simulink model "final_fuzzy_modified_fullfuzzy"  (Simulink 7.4)
settings: Solver=ode23tb  StartTime=0.0  StopTime=0.5  MaxStep=1e-5  RelTol=1e-4
undefined symbols (not defined in the file): NEWFLC1
libraries: powerlib x25, powerlib_extras x3, fuzwiz x2, powerlib_models x1, fuzblock x1
(part 1 of 2)
settings Model: Creator=Pelab  LastModifiedBy=NEC@SATYA  SimulationMode=accelerator
settings SolverCC: ZeroCrossControl=DisableAll
settings OptimizationCC: InitFltsAndDblsToZero=on
settings DebuggingCC: SaveWithParameterizedLinksMsg=none  SignalResolutionControl=TryResolveAllWithWarning  MultiTaskDSMMsg=warning  MultiTaskCondExecSysMsg=none
settings HardwareCC: TargetEndianess=LittleEndian  TargetHWDeviceType=MATLAB Host  ProdEqTarget=off
settings RTWCC: SystemTargetFile=accel.tlc  TemplateMakefile=accel_default_tmf  ProcessScript=accel_make_rtw_hook  IncludeERTFirstTime=on
settings STFCustomTargetCC: TargetFcnLib=ansi_tfl_tmw.mat  GeneratePreprocessorConditionals=Disable all  SystemTargetFile=accel.tlc

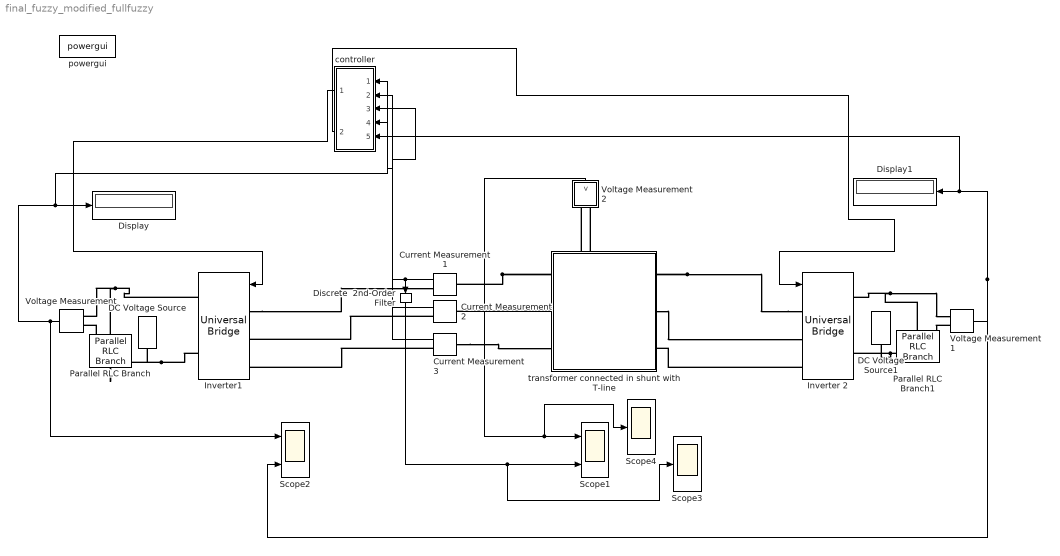
== system final_fuzzy_modified_fullfuzzy ==
  Current Measurement1 : powerlib/Measurements/Current Measurement  DialogController=POWERSYS.PowerSysDialog  SystemSampleTime=-1  PhasorSimulation=off  OutputType=Complex  PSBequivalent=0
  Current Measurement2 : powerlib/Measurements/Current Measurement  DialogController=POWERSYS.PowerSysDialog  SystemSampleTime=-1  PhasorSimulation=off  OutputType=Complex  PSBequivalent=0
  Current Measurement3 : powerlib/Measurements/Current Measurement  DialogController=POWERSYS.PowerSysDialog  SystemSampleTime=-1  PhasorSimulation=off  OutputType=Complex  PSBequivalent=0
  DC Voltage Source : powerlib/Electrical Sources/DC Voltage Source  DialogController=POWERSYS.PowerSysDialog  SystemSampleTime=-1  Amplitude=805.27  Measurements=None
  DC Voltage Source1 : powerlib/Electrical Sources/DC Voltage Source  DialogController=POWERSYS.PowerSysDialog  SystemSampleTime=-1  Amplitude=294.72  Measurements=None
  Discrete  2nd-Order Filter : powerlib_extras/Discrete  Control Blocks/Discrete  2nd-Order Filter  DialogController=POWERSYS.PowerSysDialog  SystemSampleTime=-1  FilterType=Lowpass  Fo=72  Zeta=0.707  Ts=50e-6  Initialize=off  Vac_Init=[0.8 -25 60]  Vdc_Init=-0.4  PlotResponse=off  param1=[1 500 1]
  Display : Display
      settings: Decimation=2
  Display1 : Display
  Inverter 2 : powerlib/Power Electronics/Universal Bridge  DialogController=POWERSYS.PowerSysDialog  SystemSampleTime=-1  Arms=3  SnubberResistance=1e5  SnubberCapacitance=inf  Device=Ideal Switches  Ron=1e-3  Lon=0  ForwardVoltages="[  0  0  ]"  ForwardVoltage=0  GTOparameters=[ 10e-6 , 20e-6 ]  IGBTparameters=[ 1e-6 , 2e-6 ]  Measurements=None  Measurements_2=None  converterType=Rectifier
  Inverter1 : powerlib/Power Electronics/Universal Bridge  DialogController=POWERSYS.PowerSysDialog  SystemSampleTime=-1  Arms=3  SnubberResistance=1e5  SnubberCapacitance=inf  Device=Ideal Switches  Ron=1e-3  Lon=0  ForwardVoltages="[  0  0  ]"  ForwardVoltage=0  GTOparameters=[ 10e-6 , 20e-6 ]  IGBTparameters=[ 1e-6 , 2e-6 ]  Measurements=None  Measurements_2=None  converterType=Rectifier
  Parallel RLC Branch : powerlib/Elements/Parallel RLC Branch  DialogController=POWERSYS.PowerSysDialog  PhysicalDomain=powersysdomain  SubClassName=unknown  LeftPortType=p1  RightPortType=p1  LConnTagsString=a  RConnTagsString=__new0  BranchType=RC  Resistance=1e3  Inductance=1e-3  SetiL0=off  InitialCurrent=0  Capacitance=4700e-6  Setx0=on  InitialVoltage=-805.27  Measurements=None
  Parallel RLC Branch1 : powerlib/Elements/Parallel RLC Branch  DialogController=POWERSYS.PowerSysDialog  PhysicalDomain=powersysdomain  SubClassName=unknown  LeftPortType=p1  RightPortType=p1  LConnTagsString=a  RConnTagsString=__new0  BranchType=RC  Resistance=1e3  Inductance=1e-3  SetiL0=off  InitialCurrent=0  Capacitance=4700e-6  Setx0=on  InitialVoltage=-294.72  Measurements=None
  Scope1 : Scope  NumInputPorts=2
      settings: TimeRange=0.5  YMin=-750~-100  YMax=200~40  SampleInput=on  SampleTime=1e-6
  Scope2 : Scope  NumInputPorts=2
      settings: TimeRange=0.5  YMin=0~0  YMax=1000~500  SampleInput=on  SampleTime=1e-6
  Scope3 : Scope
      settings: TimeRange=0.5  YMin=-750  YMax=200  SaveName=final_yhd_iaa  SampleInput=on  SampleTime=1e-6
  Scope4 : Scope
      settings: TimeRange=0.5  YMin=-750  YMax=200  SaveName=final_thd_Vaa  SampleInput=on  SampleTime=1e-6
  Voltage Measurement : powerlib/Measurements/Voltage Measurement  DialogController=POWERSYS.PowerSysDialog  SystemSampleTime=-1  PhasorSimulation=off  OutputType=Complex  PSBequivalent=0
  Voltage Measurement1 : powerlib/Measurements/Voltage Measurement  DialogController=POWERSYS.PowerSysDialog  SystemSampleTime=-1  PhasorSimulation=off  OutputType=Complex  PSBequivalent=0
  Voltage Measurement2 : Subsystem  AncestorBlock=powerlib/Measurements/Voltage Measurement  DialogController=POWERSYS.PowerSysDialog  mask(Voltage Measurement){PhasorSimulation=off, OutputType=Complex, PSBequivalent=0}
      mask prompts: PhasorSimulation "Phasor simulation"; OutputType "Output signal :"; PSBequivalent "Equivalent circuit"
      mask help: Ideal voltage measurement.
      mask init:
      | block = gcb;
      | powericon('psbloadfunction',block,'Measurement Block','Initialize');
      | powericon('MeasurementBlockInit',block);
      | power_initmask();
      settings: CopyFcn=powericon('psbloadfunction',gcb,'Measurement Block','UpdateGotoTag');
      mask Help: web(psbhelp);
      mask StyleString: checkbox,popup(Complex|Real-Imag|Magnitude-Angle|Magnitude),edit
  controller : Subsystem
  powergui : powerlib/powergui  SystemSampleTime=-1  SimulationMode=Continuous  SampleTime=0  frequency=60  SPID=off  DisableSnubberDevices=off  DisableRonSwitches=off  DisableVfSwitches=off  SwTol=0  Interpol=off  frequencyindice=50  echomessages=off  HookPort=off  DisplayEquations=off  FunctionMessages=off  EnableUseOfTLC=off  x0status=blocks  RestoreLinks=warning  Frange=[0:2:500]  Ylog=off  Xlog=on  ShowGrid=off  save=off  variable=ZData  structure=final_thd  ZoomFFT=off  StartTime=0.08  cycles=1  DisplayStyle=1  fundamental=50  FreqAxis=on  MaxFrequency=2500  frequencyindicesteady=1  RmsSteady=1  display=off  Ts=0  methode=off
  transformer connected in shunt with T-line : Subsystem
  wires:
  Voltage Measurement1/1 -> Display1/1, controller/5(In5), Scope2/2
  Voltage Measurement/1 -> Display/1, controller/4(In4), Scope2/1
  Current Measurement1/1 -> controller/1(In1), Discrete  2nd-Order Filter/1
  Current Measurement2/1 -> controller/2(In2)
  Current Measurement3/1 -> controller/3(In3)
  controller/1(Out1) -> Inverter1/1
  controller/2(Out2) -> Inverter 2/1
  Voltage Measurement2/1(v) -> Scope1/1, Scope4/1
  Discrete  2nd-Order Filter/1 -> Scope1/2, Scope3/1
  connections:
  Inverter1/RConn2 -- Parallel RLC Branch/LConn1 -- Voltage Measurement/LConn2 -- DC Voltage Source/LConn1
  Parallel RLC Branch1/LConn1 -- Voltage Measurement1/LConn2 -- Inverter 2/RConn2 -- DC Voltage Source1/LConn1
  Inverter 2/LConn1 -- transformer connected in shunt with T-line/LConn1 -- Voltage Measurement2/LConn2
  transformer connected in shunt with T-line/LConn2 -- Inverter 2/LConn2
  Inverter 2/LConn3 -- transformer connected in shunt with T-line/LConn3
  Parallel RLC Branch/RConn1 -- Inverter1/RConn1 -- Voltage Measurement/LConn1
  Parallel RLC Branch1/RConn1 -- Inverter 2/RConn1 -- Voltage Measurement1/LConn1
  transformer connected in shunt with T-line/RConn1 -- Current Measurement1/LConn1 -- Voltage Measurement2/LConn1
  Inverter1/LConn1 -- Current Measurement1/RConn1
  transformer connected in shunt with T-line/RConn2 -- Current Measurement2/LConn1
  Current Measurement2/RConn1 -- Inverter1/LConn2
  Current Measurement3/LConn1 -- transformer connected in shunt with T-line/RConn3
  Current Measurement3/RConn1 -- Inverter1/LConn3

== system final_fuzzy_modified_fullfuzzy/Voltage Measurement2 ==
  Discrete  2nd-Order Filter : powerlib_extras/Discrete  Control Blocks/Discrete  2nd-Order Filter  DialogController=POWERSYS.PowerSysDialog  SystemSampleTime=-1  FilterType=Lowpass  Fo=2000  Zeta=0.707  Ts=50e-6  Initialize=off  Vac_Init=[0.8 -25 60]  Vdc_Init=-0.4  PlotResponse=off  param1=[1 500 1]
  VoltageMeasurement : PMComponent  PhysicalDomain=powersysdomain  LeftPortType=p1  RightPortType=p1  LConnTagsString=+  RConnTagsString=-
      mask Type: InnerPowersysBlock
  do not delete this gain : Gain  ParameterDataType=sfix(16)  ParameterScaling=2^0  OutDataType=sfix(16)  OutScaling=2^0
  model : powerlib_models/Continuous/Measurement  SystemSampleTime=-1
  + : PMIOPort  Port=1  Side=Left
  - : PMIOPort  Port=2  Side=Left
  v : Outport  OutDataType=sfix(16)  OutScaling=2^0  InitialOutput=0
  wires:
  do not delete this gain/1 -> Discrete  2nd-Order Filter/1
  model/1 -> do not delete this gain/1
  [tpa3b51407_3347_4229_bbae_ba988a9393db] -> model/1
  Discrete  2nd-Order Filter/1 -> v/1
  connections:
  -/RConn1 -- VoltageMeasurement/RConn1
  +/RConn1 -- VoltageMeasurement/LConn1

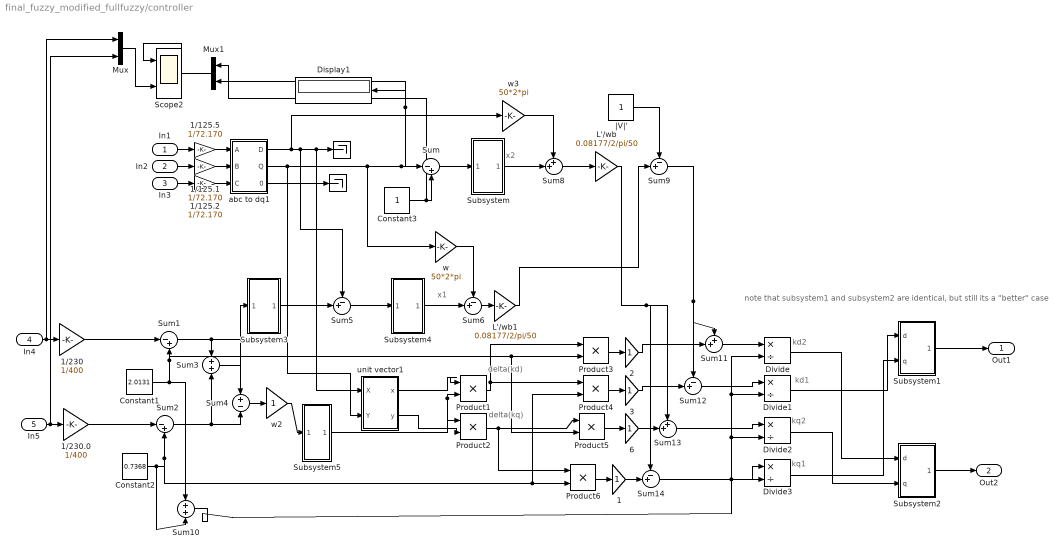
== system final_fuzzy_modified_fullfuzzy/controller ==
  note: x1
  note: x2
  note: delta(kd)
  note: delta(kq)
  note: kq2
  note: kd2
  note: kd1
  note: kq1
  note: note that subsystem1 and subsystem2 are identical,
      | but still its a "better" case
  In1 : Inport  OutDataType=sfix(16)  OutScaling=2^0
  In2 : Inport  Port=2  OutDataType=sfix(16)  OutScaling=2^0
  In3 : Inport  Port=3  OutDataType=sfix(16)  OutScaling=2^0
  In4 : Inport  Port=4  OutDataType=sfix(16)  OutScaling=2^0
  In5 : Inport  Port=5  OutDataType=sfix(16)  OutScaling=2^0
  " " : Terminator
  "  " : Terminator
  {1..3,6} (4 alike) : Gain  ParameterDataType=sfix(16)  ParameterScaling=2^0  OutDataType=sfix(16)  OutScaling=2^0
  1/125.1 : Gain  Gain=1/72.170  ParameterDataType=sfix(16)  ParameterScaling=2^0  OutDataType=sfix(16)  OutScaling=2^0
  1/125.2 : Gain  Gain=1/72.170  ParameterDataType=sfix(16)  ParameterScaling=2^0  OutDataType=sfix(16)  OutScaling=2^0
  1/125.5 : Gain  Gain=1/72.170  ParameterDataType=sfix(16)  ParameterScaling=2^0  OutDataType=sfix(16)  OutScaling=2^0
  1/230 : Gain  Gain=1/400  ParameterDataType=sfix(16)  ParameterScaling=2^0  OutDataType=sfix(16)  OutScaling=2^0
  1/230.0 : Gain  Gain=1/400  ParameterDataType=sfix(16)  ParameterScaling=2^0  OutDataType=sfix(16)  OutScaling=2^0
  Constant1 : Constant  Value=2.0131  OutDataType=sfix(16)  OutScaling=2^0
  Constant2 : Constant  Value=0.7368  OutDataType=sfix(16)  OutScaling=2^0
  Constant3 : Constant  OutDataType=sfix(16)  OutScaling=2^0
  Display1 : Display
  Divide{,1..3} (4 alike) : Product  Inputs=*/  OutDataType=sfix(16)  OutScaling=2^-10
  L'/wb : Gain  Gain=0.08177/2/pi/50  ParameterDataType=sfix(16)  ParameterScaling=2^0  OutDataType=sfix(16)  OutScaling=2^0
  L'/wb1 : Gain  Gain=0.08177/2/pi/50  ParameterDataType=sfix(16)  ParameterScaling=2^0  OutDataType=sfix(16)  OutScaling=2^0
  Mux : Mux  Inputs=2
  Mux1 : Mux  Inputs=2
  Product{1..6} (6 alike) : Product  OutDataType=sfix(16)  OutScaling=2^0  RndMeth=Zero
  Scope2 : Scope  NumInputPorts=2
      settings: TimeRange=0.03256302521008403  YMin=1~275  YMax=1.85~825  SaveName=ScopeData2  SampleTime=1e-6
  Subsystem : Subsystem
  Subsystem1 : Subsystem
  Subsystem2 : Subsystem
  Subsystem3 : Subsystem
  Subsystem4 : Subsystem
  Subsystem5 : Subsystem
  Sum : Sum  Inputs=|-+  OutDataType=sfix(16)  OutScaling=2^0
  Sum1 : Sum  Inputs=|-+  OutDataType=sfix(16)  OutScaling=2^0
  Sum10 : Sum  OutDataType=sfix(16)  OutScaling=2^0
  Sum11 : Sum  Inputs=++|  OutDataType=sfix(16)  OutScaling=2^0
  Sum{5..6,9,12,14} (5 alike) : Sum  Inputs=-+|  OutDataType=sfix(16)  OutScaling=2^0
  Sum13 : Sum  Inputs=++|  OutDataType=sfix(16)  OutScaling=2^0
  Sum2 : Sum  Inputs=|-+  OutDataType=sfix(16)  OutScaling=2^0
  Sum3 : Sum  OutDataType=sfix(16)  OutScaling=2^0
  Sum4 : Sum  Inputs=+-  OutDataType=sfix(16)  OutScaling=2^0
  Sum8 : Sum  Inputs=++|  OutDataType=sfix(16)  OutScaling=2^0
  abc to dq1 : Subsystem
  unit vector1 : Subsystem
  w : Gain  Gain=50*2*pi  ParameterDataType=sfix(16)  ParameterScaling=2^0  OutDataType=sfix(16)  OutScaling=2^0
  w2 : Gain  ParameterDataType=sfix(16)  ParameterScaling=2^0  OutDataType=sfix(16)  OutScaling=2^0
  w3 : Gain  Gain=50*2*pi  ParameterDataType=sfix(16)  ParameterScaling=2^0  OutDataType=sfix(16)  OutScaling=2^0
  |V|' : Constant  OutDataType=sfix(16)  OutScaling=2^0
  Out1 : Outport  OutDataType=sfix(16)  OutScaling=2^0
  Out2 : Outport  Port=2  OutDataType=sfix(16)  OutScaling=2^0
  wires:
  Constant3/1 -> Sum/2, Mux1/1
  abc to dq1/1(D) -> " "/1, unit vector1/1(X), Sum5/1, w3/1
  abc to dq1/3(0) -> "  "/1
  In1/1 -> 1/125.5/1
  In2/1 -> 1/125.1/1
  In3/1 -> 1/125.2/1
  In4/1 -> 1/230/1, Mux/1
  In5/1 -> 1/230.0/1, Mux/2
  Constant1/1 -> Sum1/2, Product3/2, Product5/2, Sum10/1
  Constant2/1 -> Sum2/2, Product6/2, Product4/2, Sum10/2
  Sum/1 -> Subsystem/1(In3)
  Sum1/1 -> Sum3/1, Sum4/1
  Sum2/1 -> Sum3/2, Sum4/2
  abc to dq1/2(Q) -> w/1, Sum/1, Display1/1, Mux1/2, unit vector1/2(Y)
  Sum5/1 -> Subsystem4/1(In3)
  Sum4/1 -> w2/1
  Sum3/1 -> Subsystem3/1(In3)
  Product1/1 -> Product4/1, Product3/1
  Product2/1 -> Product5/1, Product6/1
  |V|'/1 -> Sum9/1
  Sum9/1 -> Sum11/1, Sum12/1
  Sum11/1 -> Divide/1
  Sum10/1 -> Divide/2, Divide1/2, Divide2/2, Divide3/2
  Sum12/1 -> Divide1/1
  Product5/1 -> 6/1
  Sum13/1 -> Divide2/1
  Product6/1 -> 1/1
  Sum14/1 -> Divide3/1
  Sum6/1 -> L'/wb1/1
  unit vector1/1(x) -> Product1/1
  unit vector1/2(y) -> Product2/2
  Product3/1 -> 2/1
  Product4/1 -> 3/1
  Subsystem/1(Out1) -> Sum8/2
  Subsystem4/1(Out1) -> Sum6/2
  L'/wb/1 -> Sum13/1, Sum14/1
  L'/wb1/1 -> Sum9/2
  1/1 -> Sum14/2
  6/1 -> Sum13/2
  2/1 -> Sum11/2
  3/1 -> Sum12/2
  Sum8/1 -> L'/wb/1
  w2/1 -> Subsystem5/1(In3)
  Subsystem1/1(pwm) -> Out1/1
  Subsystem2/1(pwm) -> Out2/1
  Divide/1 -> Subsystem2/1(d)
  Divide1/1 -> Subsystem1/1(d)
  Divide2/1 -> Subsystem2/2(q)
  Divide3/1 -> Subsystem1/2(q)
  1/230/1 -> Sum1/1
  1/230.0/1 -> Sum2/1
  1/125.5/1 -> abc to dq1/1(A)
  1/125.1/1 -> abc to dq1/2(B)
  1/125.2/1 -> abc to dq1/3(C)
  Subsystem3/1(Out1) -> Sum5/2
  Mux/1 -> Scope2/2
  Mux1/1 -> Scope2/1
  w3/1 -> Sum8/1
  w/1 -> Sum6/1
  Subsystem5/1(Out1) -> Product1/2, Product2/1

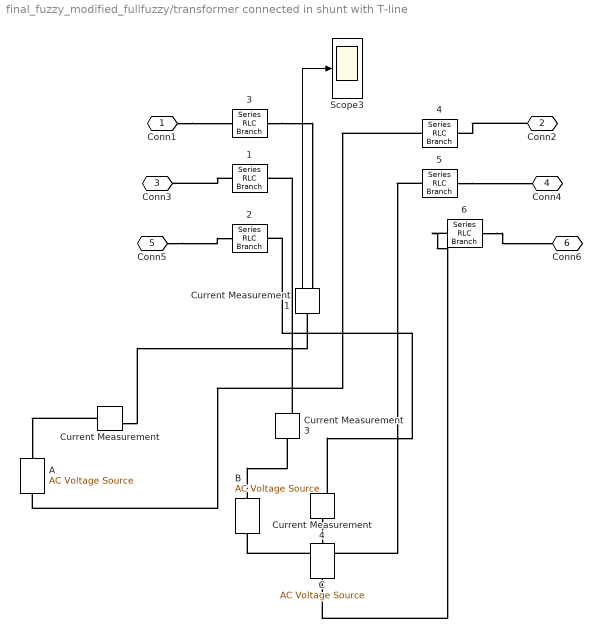
== system final_fuzzy_modified_fullfuzzy/transformer connected in shunt with T-line ==
    {1..6} (6 alike) : powerlib/Elements/Series RLC Branch  DialogController=POWERSYS.PowerSysDialog  PhysicalDomain=powersysdomain  SubClassName=unknown  LeftPortType=p1  RightPortType=p1  LConnTagsString=__new0  RConnTagsString=__new0  BranchType=RL  Resistance=0.6  Inductance=(2.5e-3)/2  SetiL0=off  InitialCurrent=0  Capacitance=1e-6  Setx0=off  InitialVoltage=0  Measurements=None
  A : powerlib/Electrical Sources/AC Voltage Source  DialogController=POWERSYS.PowerSysDialog  SystemSampleTime=-1  Amplitude=400*1.414  Phase=0  Frequency=50  SampleTime=0  Measurements=None
  B : powerlib/Electrical Sources/AC Voltage Source  DialogController=POWERSYS.PowerSysDialog  SystemSampleTime=-1  Amplitude=400*1.414  Phase=-120  Frequency=50  SampleTime=0  Measurements=None
  C : powerlib/Electrical Sources/AC Voltage Source  DialogController=POWERSYS.PowerSysDialog  SystemSampleTime=-1  Amplitude=400*1.414  Phase=-240  Frequency=50  SampleTime=0  Measurements=None
  Current Measurement{,1,3..4} (4 alike) : powerlib/Measurements/Current Measurement  DialogController=POWERSYS.PowerSysDialog  SystemSampleTime=-1  PhasorSimulation=off  OutputType=Complex  PSBequivalent=0
  Scope3 : Scope
      settings: TimeRange=0.5  YMin=-100  YMax=100  SaveName=i1  SampleInput=on  SampleTime=1e-6
  Conn1 : PMIOPort  Port=1  Side=Right
  Conn2 : PMIOPort  Port=2  Side=Left
  Conn3 : PMIOPort  Port=3  Side=Right
  Conn4 : PMIOPort  Port=4  Side=Left
  Conn5 : PMIOPort  Port=5  Side=Right
  Conn6 : PMIOPort  Port=6  Side=Left
  wires:
  Current Measurement1/1 -> Scope3/1
  connections:
  Conn1/RConn1 -- "  3"/RConn1
  "  1"/RConn1 -- Conn3/RConn1
  "  5"/LConn1 -- Conn4/RConn1
  Conn5/RConn1 -- "  2"/RConn1
  "  6"/LConn1 -- Conn6/RConn1
  Current Measurement/RConn1 -- Current Measurement1/LConn1
  "  4"/RConn1 -- A/LConn1
  "  3"/LConn1 -- Current Measurement1/RConn1
  Current Measurement4/RConn1 -- "  2"/LConn1
  Current Measurement3/RConn1 -- "  1"/LConn1
  Conn2/RConn1 -- "  4"/LConn1
  Current Measurement/LConn1 -- A/RConn1
  B/RConn1 -- Current Measurement3/LConn1
  "  5"/RConn1 -- B/LConn1
  Current Measurement4/LConn1 -- C/RConn1
  "  6"/RConn1 -- C/LConn1

== system final_fuzzy_modified_fullfuzzy/controller/Subsystem ==
  In3 : Inport
  Derivative : Derivative
  Fuzzy Logic  Controller : fuzblock/Fuzzy Logic  Controller  SystemSampleTime=-1  fis=NEWFLC1
  Mux2 : Mux  Inputs=2
  Out1 : Outport
  wires:
  Mux2/1 -> Fuzzy Logic  Controller/1
  In3/1 -> Mux2/1, Derivative/1
  Fuzzy Logic  Controller/1 -> Out1/1
  Derivative/1 -> Mux2/2

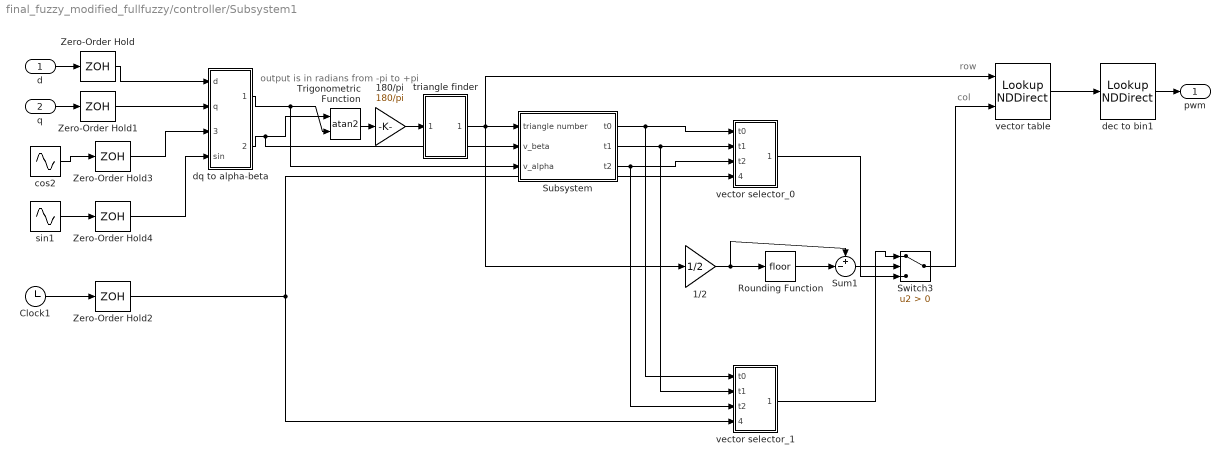
== system final_fuzzy_modified_fullfuzzy/controller/Subsystem1 ==
  note: output is in radians from -pi to +pi
  note: col
  note: row
  d : Inport  OutDataType=sfix(16)  OutScaling=2^0
  q : Inport  Port=2  OutDataType=sfix(16)  OutScaling=2^0
  1/2 : Gain  Gain=1/2  ParameterDataType=sfix(16)  ParameterScaling=2^0  OutDataType=sfix(16)  OutScaling=2^0
  180/pi : Gain  Gain=180/pi  ParameterDataType=sfix(16)  ParameterScaling=2^0  OutDataType=sfix(16)  OutScaling=2^0
  Clock1 : Clock
      settings: Decimation=10
  Rounding Function : Rounding
  Subsystem : Subsystem
  Sum1 : Sum  Inputs=+-|  OutDataType=sfix(16)  OutScaling=2^0
  Switch3 : Switch  Criteria=u2 > Threshold
  Trigonometric Function : Trigonometry  Operator=atan2
  Zero-Order Hold{,1..4} (5 alike) : ZeroOrderHold  SampleTime=(20e-3)/18
  cos2 : Sin  Amplitude=1  Bias=0  Frequency=50*2*pi  Phase=pi/2  Samples=10  SampleTime=0  Offset=0
  dec to bin1 : LookupNDDirect  InputsSelectThisObjectFromTable=Column  Table=[0 1 1 0 0 0 1 1; 1 0 0 1 1 1 0 0; 0 0 1 1 1 0 0 1; 1 1 0 0 0 1 1 0; 0 0 0 0 1 1 1 1; 1 1 1 1 0 0 0 0]
  dq to alpha-beta : Subsystem
  sin1 : Sin  Amplitude=1  Bias=0  Frequency=50*2*pi  Phase=0  Samples=10  SampleTime=0  Offset=0
  triangle finder : Subsystem
  vector selector_0 : Subsystem
  vector selector_1 : Subsystem
  vector table : LookupNDDirect  Table=[0 5 6 7 6 5 0; 0 1 6 7 6 1 0; 0 1 2 7 2 1 0; 0 3 2 7 2 3 0; 0 3 4 7 4 3 0; 0 5 4 7 4 5 0]
  pwm : Outport  OutDataType=sfix(16)  OutScaling=2^0
  wires:
  dq to alpha-beta/2(beta) -> Trigonometric Function/1, Subsystem/2(v_beta)
  dq to alpha-beta/1(alpha) -> Trigonometric Function/2, Subsystem/3(v_alpha)
  Trigonometric Function/1 -> 180/pi/1
  180/pi/1 -> triangle finder/1(In1)
  triangle finder/1(Out1) -> Subsystem/1(triangle number), vector table/1, 1/2/1
  Zero-Order Hold/1 -> dq to alpha-beta/1(d)
  Zero-Order Hold1/1 -> dq to alpha-beta/2(q)
  Clock1/1 -> Zero-Order Hold2/1
  Zero-Order Hold2/1 -> vector selector_0/4(hold_time), vector selector_1/4(hold_time)
  vector table/1 -> dec to bin1/1
  dec to bin1/1 -> pwm/1
  d/1 -> Zero-Order Hold/1
  q/1 -> Zero-Order Hold1/1
  cos2/1 -> Zero-Order Hold3/1
  Zero-Order Hold3/1 -> dq to alpha-beta/3(cos)
  sin1/1 -> Zero-Order Hold4/1
  Zero-Order Hold4/1 -> dq to alpha-beta/4(sin)
  1/2/1 -> Rounding Function/1, Sum1/1
  Rounding Function/1 -> Sum1/2
  Sum1/1 -> Switch3/2
  Subsystem/1(t0) -> vector selector_0/1(t0), vector selector_1/1(t0)
  Subsystem/2(t1) -> vector selector_0/2(t1), vector selector_1/2(t1)
  Subsystem/3(t2) -> vector selector_0/3(t2), vector selector_1/3(t2)
  vector selector_0/1(Out1) -> Switch3/3
  Switch3/1 -> vector table/2
  vector selector_1/1(Out1) -> Switch3/1

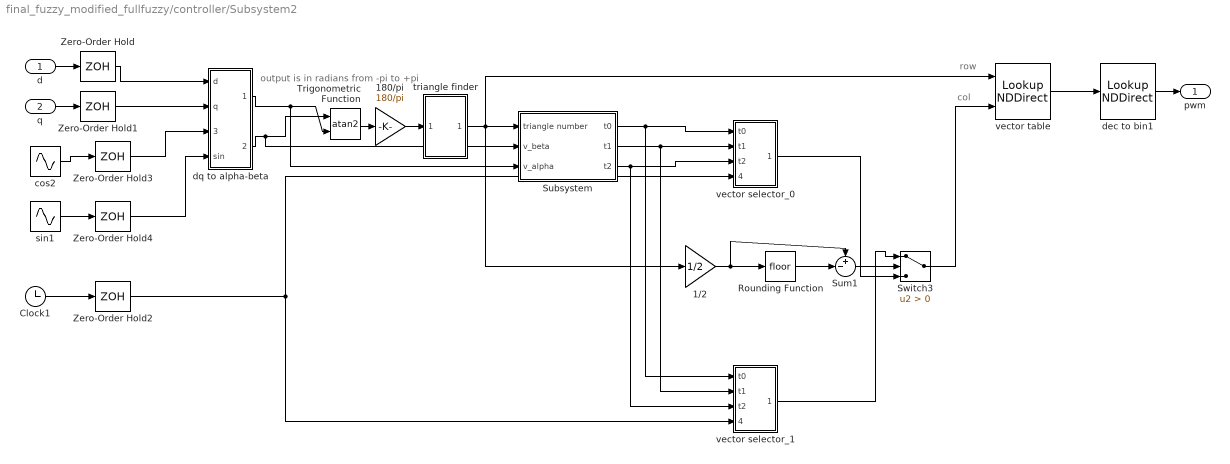
== system final_fuzzy_modified_fullfuzzy/controller/Subsystem2 ==
  note: row
  note: col
  note: output is in radians from -pi to +pi
  d : Inport  OutDataType=sfix(16)  OutScaling=2^0
  q : Inport  Port=2  OutDataType=sfix(16)  OutScaling=2^0
  1/2 : Gain  Gain=1/2  ParameterDataType=sfix(16)  ParameterScaling=2^0  OutDataType=sfix(16)  OutScaling=2^0
  180/pi : Gain  Gain=180/pi  ParameterDataType=sfix(16)  ParameterScaling=2^0  OutDataType=sfix(16)  OutScaling=2^0
  Clock1 : Clock
      settings: Decimation=10
  Rounding Function : Rounding
  Subsystem : Subsystem
  Sum1 : Sum  Inputs=+-|  OutDataType=sfix(16)  OutScaling=2^0
  Switch3 : Switch  Criteria=u2 > Threshold
  Trigonometric Function : Trigonometry  Operator=atan2
  Zero-Order Hold{,1..4} (5 alike) : ZeroOrderHold  SampleTime=(20e-3)/18
  cos2 : Sin  Amplitude=1  Bias=0  Frequency=50*2*pi  Phase=pi/2  Samples=10  SampleTime=0  Offset=0
  dec to bin1 : LookupNDDirect  InputsSelectThisObjectFromTable=Column  Table=[0 1 1 0 0 0 1 1; 1 0 0 1 1 1 0 0; 0 0 1 1 1 0 0 1; 1 1 0 0 0 1 1 0; 0 0 0 0 1 1 1 1; 1 1 1 1 0 0 0 0]
  dq to alpha-beta : Subsystem
  sin1 : Sin  Amplitude=1  Bias=0  Frequency=50*2*pi  Phase=0  Samples=10  SampleTime=0  Offset=0
  triangle finder : Subsystem
  vector selector_0 : Subsystem
  vector selector_1 : Subsystem
  vector table : LookupNDDirect  Table=[0 5 6 7 6 5 0; 0 1 6 7 6 1 0; 0 1 2 7 2 1 0; 0 3 2 7 2 3 0; 0 3 4 7 4 3 0; 0 5 4 7 4 5 0]
  pwm : Outport  OutDataType=sfix(16)  OutScaling=2^0
  wires:
  vector selector_1/1(Out1) -> Switch3/1
  Switch3/1 -> vector table/2
  vector selector_0/1(Out1) -> Switch3/3
  Subsystem/3(t2) -> vector selector_1/3(t2), vector selector_0/3(t2)
  Subsystem/2(t1) -> vector selector_1/2(t1), vector selector_0/2(t1)
  Subsystem/1(t0) -> vector selector_1/1(t0), vector selector_0/1(t0)
  Sum1/1 -> Switch3/2
  Rounding Function/1 -> Sum1/2
  1/2/1 -> Sum1/1, Rounding Function/1
  Zero-Order Hold4/1 -> dq to alpha-beta/4(sin)
  sin1/1 -> Zero-Order Hold4/1
  Zero-Order Hold3/1 -> dq to alpha-beta/3(cos)
  cos2/1 -> Zero-Order Hold3/1
  q/1 -> Zero-Order Hold1/1
  d/1 -> Zero-Order Hold/1
  dec to bin1/1 -> pwm/1
  vector table/1 -> dec to bin1/1
  Zero-Order Hold2/1 -> vector selector_1/4(hold_time), vector selector_0/4(hold_time)
  Clock1/1 -> Zero-Order Hold2/1
  Zero-Order Hold1/1 -> dq to alpha-beta/2(q)
  Zero-Order Hold/1 -> dq to alpha-beta/1(d)
  triangle finder/1(Out1) -> 1/2/1, vector table/1, Subsystem/1(triangle number)
  180/pi/1 -> triangle finder/1(In1)
  Trigonometric Function/1 -> 180/pi/1
  dq to alpha-beta/1(alpha) -> Subsystem/3(v_alpha), Trigonometric Function/2
  dq to alpha-beta/2(beta) -> Subsystem/2(v_beta), Trigonometric Function/1

== system final_fuzzy_modified_fullfuzzy/controller/Subsystem3 ==
  In3 : Inport
  Derivative : Derivative
  Fuzzy Logic  Controller : Subsystem  AncestorBlock="fuzblock/Fuzzy Logic  Controller"  mask(FIS){fis=NEWFLC1}
      mask prompts: fis "FIS file or structure:"
      mask help: FIS
      mask init:
      | fis = fuzblockmask(gcb,fis);
      mask Help: helpview([docroot '\toolbox\fuzzy\fuzzylogiccontroller.html'])
      mask Display: plot(0, -0.3, 6, -0.3, 0, 1.2, 6, 1.2, [0 6], [0 0], [1 2 3],[0 1 0],[2 3 4],[0 1 0],[3 4 5],[0 1 0])
  Mux2 : Mux  Inputs=2
  Out1 : Outport
  wires:
  Derivative/1 -> Mux2/2
  Fuzzy Logic  Controller/1(Out1) -> Out1/1
  In3/1 -> Derivative/1, Mux2/1
  Mux2/1 -> Fuzzy Logic  Controller/1(In1)

== system final_fuzzy_modified_fullfuzzy/controller/Subsystem4 ==
  In3 : Inport
  Derivative : Derivative
  Fuzzy Logic  Controller : Subsystem  AncestorBlock="fuzblock/Fuzzy Logic  Controller"  mask(FIS){fis=NEWFLC1}
      mask prompts: fis "FIS file or structure:"
      mask help: FIS
      mask init:
      | fis = fuzblockmask(gcb,fis);
      mask Help: helpview([docroot '\toolbox\fuzzy\fuzzylogiccontroller.html'])
      mask Display: plot(0, -0.3, 6, -0.3, 0, 1.2, 6, 1.2, [0 6], [0 0], [1 2 3],[0 1 0],[2 3 4],[0 1 0],[3 4 5],[0 1 0])
  Mux2 : Mux  Inputs=2
  Out1 : Outport
  wires:
  Mux2/1 -> Fuzzy Logic  Controller/1(In1)
  In3/1 -> Mux2/1, Derivative/1
  Fuzzy Logic  Controller/1(Out1) -> Out1/1
  Derivative/1 -> Mux2/2

== system final_fuzzy_modified_fullfuzzy/controller/Subsystem5 ==
  In3 : Inport
  Derivative : Derivative
  Fuzzy Logic  Controller : Subsystem  AncestorBlock="fuzblock/Fuzzy Logic  Controller"  mask(FIS){fis=NEWFLC1}
      mask prompts: fis "FIS file or structure:"
      mask help: FIS
      mask init:
      | fis = fuzblockmask(gcb,fis);
      mask Help: helpview([docroot '\toolbox\fuzzy\fuzzylogiccontroller.html'])
      mask Display: plot(0, -0.3, 6, -0.3, 0, 1.2, 6, 1.2, [0 6], [0 0], [1 2 3],[0 1 0],[2 3 4],[0 1 0],[3 4 5],[0 1 0])
  Mux2 : Mux  Inputs=2
  Out1 : Outport
  wires:
  Mux2/1 -> Fuzzy Logic  Controller/1(In1)
  In3/1 -> Mux2/1, Derivative/1
  Fuzzy Logic  Controller/1(Out1) -> Out1/1
  Derivative/1 -> Mux2/2

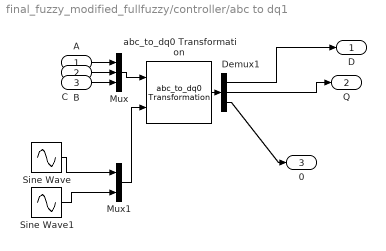
== system final_fuzzy_modified_fullfuzzy/controller/abc to dq1 ==
  A : Inport  OutDataType=sfix(16)  OutScaling=2^0
  B : Inport  Port=2  OutDataType=sfix(16)  OutScaling=2^0
  C : Inport  Port=3  OutDataType=sfix(16)  OutScaling=2^0
  Demux1 : Demux  Outputs=3
  Mux : Mux  Inputs=3
  Mux1 : Mux  Inputs=2
  Sine Wave : Sin  Amplitude=1  Bias=0  Frequency=50*2*pi  Phase=0  Samples=10  SampleTime=0  Offset=0
  Sine Wave1 : Sin  Amplitude=1  Bias=0  Frequency=50*2*pi  Phase=pi/2  Samples=10  SampleTime=0  Offset=0
  abc_to_dq0 Transformation : powerlib_extras/Measurements/abc_to_dq0 Transformation  DialogController=POWERSYS.PowerSysDialog  SystemSampleTime=-1
  D : Outport  OutDataType=sfix(16)  OutScaling=2^0
  Q : Outport  Port=2  OutDataType=sfix(16)  OutScaling=2^0
  0 : Outport  Port=3  OutDataType=sfix(16)  OutScaling=2^0
  wires:
  Demux1/3 -> 0/1
  C/1 -> Mux/3
  B/1 -> Mux/2
  A/1 -> Mux/1
  Mux/1 -> abc_to_dq0 Transformation/1
  Sine Wave/1 -> Mux1/1
  Sine Wave1/1 -> Mux1/2
  Mux1/1 -> abc_to_dq0 Transformation/2
  abc_to_dq0 Transformation/1 -> Demux1/1
  Demux1/1 -> D/1
  Demux1/2 -> Q/1

== system final_fuzzy_modified_fullfuzzy/controller/unit vector1 ==
  X : Inport  OutDataType=sfix(16)  OutScaling=2^0
  Y : Inport  Port=2  OutDataType=sfix(16)  OutScaling=2^0
  Add : Sum  OutDataType=sfix(16)  OutScaling=2^-10
  Divide : Product  Inputs=*/  OutDataType=sfix(16)  OutScaling=2^-10
  Divide1 : Product  Inputs=*/  OutDataType=sfix(16)  OutScaling=2^-10
  Math Function : Math  Operator=sqrt  OutDataType=sfix(16)  OutScaling=2^0  SaturateOnIntegerOverflow=on
  Product : Product  OutDataType=sfix(16)  OutScaling=2^0  RndMeth=Zero
  Product1 : Product  OutDataType=sfix(16)  OutScaling=2^0  RndMeth=Zero
  Saturation : Saturate  UpperLimit=inf  LowerLimit=0.0001
  x : Outport  OutDataType=sfix(16)  OutScaling=2^0
  y : Outport  Port=2  OutDataType=sfix(16)  OutScaling=2^0
  wires:
  Saturation/1 -> Divide1/2, Divide/2
  Divide1/1 -> y/1
  Divide/1 -> x/1
  Math Function/1 -> Saturation/1
  Add/1 -> Math Function/1
  Y/1 -> Divide1/1, Product1/2, Product1/1
  X/1 -> Divide/1, Product/2, Product/1
  Product1/1 -> Add/2
  Product/1 -> Add/1

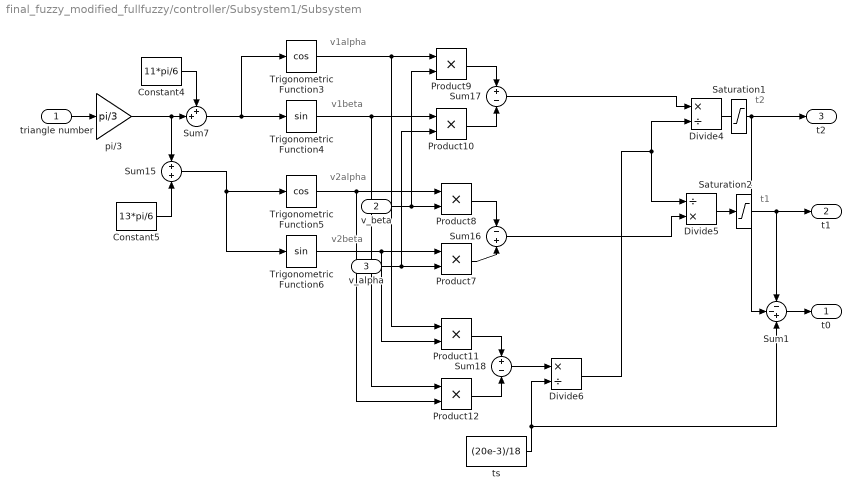
== system final_fuzzy_modified_fullfuzzy/controller/Subsystem1/Subsystem ==
  note: v1alpha
  note: v1beta
  note: v2alpha
  note: v2beta
  note: t1
  note: t2
  triangle number : Inport  OutDataType=sfix(16)  OutScaling=2^0
  v_beta : Inport  Port=2  OutDataType=sfix(16)  OutScaling=2^0
  v_alpha : Inport  Port=3  OutDataType=sfix(16)  OutScaling=2^0
  Constant4 : Constant  Value=11*pi/6  OutDataType=sfix(16)  OutScaling=2^0
  Constant5 : Constant  Value=13*pi/6  OutDataType=sfix(16)  OutScaling=2^0
  Divide4 : Product  Inputs=*/  OutDataType=sfix(16)  OutScaling=2^-10
  Divide5 : Product  Inputs=/*  OutDataType=sfix(16)  OutScaling=2^-10
  Divide6 : Product  Inputs=*/  OutDataType=sfix(16)  OutScaling=2^-10
  Product{7..12} (6 alike) : Product  OutDataType=sfix(16)  OutScaling=2^0  RndMeth=Zero
  Saturation1 : Saturate  UpperLimit=inf  LowerLimit=0
  Saturation2 : Saturate  UpperLimit=inf  LowerLimit=0
  Sum1 : Sum  Inputs=--+  OutDataType=sfix(16)  OutScaling=2^0
  Sum15 : Sum  OutDataType=sfix(16)  OutScaling=2^0
  Sum16 : Sum  Inputs=-+  OutDataType=sfix(16)  OutScaling=2^0
  Sum17 : Sum  Inputs=+-  OutDataType=sfix(16)  OutScaling=2^0
  Sum18 : Sum  Inputs=+-  OutDataType=sfix(16)  OutScaling=2^0
  Sum7 : Sum  Inputs=++|  OutDataType=sfix(16)  OutScaling=2^0
  Trigonometric Function3 : Trigonometry  Operator=cos
  Trigonometric Function4 : Trigonometry
  Trigonometric Function5 : Trigonometry  Operator=cos
  Trigonometric Function6 : Trigonometry
  pi/3 : Gain  Gain=pi/3  ParameterDataType=sfix(16)  ParameterScaling=2^0  OutDataType=sfix(16)  OutScaling=2^0
  ts : Constant  Value=(20e-3)/18  OutDataType=sfix(16)  OutScaling=2^0
  t0 : Outport  OutDataType=sfix(16)  OutScaling=2^0
  t1 : Outport  Port=2  OutDataType=sfix(16)  OutScaling=2^0
  t2 : Outport  Port=3  OutDataType=sfix(16)  OutScaling=2^0
  wires:
  Sum7/1 -> Trigonometric Function3/1, Trigonometric Function4/1
  Constant4/1 -> Sum7/1
  pi/3/1 -> Sum7/2, Sum15/1
  Constant5/1 -> Sum15/2
  Trigonometric Function5/1 -> Product8/1, Product12/2
  Trigonometric Function6/1 -> Product7/1, Product11/2
  Sum15/1 -> Trigonometric Function5/1, Trigonometric Function6/1
  Product7/1 -> Sum16/2
  Product8/1 -> Sum16/1
  Sum16/1 -> Divide5/2
  Trigonometric Function3/1 -> Product9/1, Product11/1
  Trigonometric Function4/1 -> Product10/1, Product12/1
  Product9/1 -> Sum17/1
  Product10/1 -> Sum17/2
  Sum17/1 -> Divide4/1
  Product11/1 -> Sum18/1
  Product12/1 -> Sum18/2
  Sum18/1 -> Divide6/1
  Divide6/1 -> Divide4/2, Divide5/1
  ts/1 -> Divide6/2, Sum1/3
  v_beta/1 -> Product8/2, Product9/2
  v_alpha/1 -> Product7/2, Product10/2
  Divide4/1 -> Sum1/2, t2/1
  triangle number/1 -> pi/3/1
  Divide5/1 -> Saturation2/1
  Sum1/1 -> t0/1
  Saturation2/1 -> t1/1, Sum1/1

== system final_fuzzy_modified_fullfuzzy/controller/Subsystem1/dq to alpha-beta ==
  d : Inport  OutDataType=sfix(16)  OutScaling=2^0
  q : Inport  Port=2  OutDataType=sfix(16)  OutScaling=2^0
  cos : Inport  Port=3  OutDataType=sfix(16)  OutScaling=2^0
  sin : Inport  Port=4  OutDataType=sfix(16)  OutScaling=2^0
  Product{,1..3} (4 alike) : Product  OutDataType=sfix(16)  OutScaling=2^0  RndMeth=Zero
  Sum : Sum  Inputs=+-  OutDataType=sfix(16)  OutScaling=2^0
  Sum1 : Sum  OutDataType=sfix(16)  OutScaling=2^0
  alpha : Outport  OutDataType=sfix(16)  OutScaling=2^0
  beta : Outport  Port=2  OutDataType=sfix(16)  OutScaling=2^0
  wires:
  d/1 -> Product/1, Product2/1
  q/1 -> Product1/2, Product3/1
  Product/1 -> Sum/1
  Product1/1 -> Sum/2
  Sum/1 -> alpha/1
  Product2/1 -> Sum1/1
  Product3/1 -> Sum1/2
  Sum1/1 -> beta/1
  cos/1 -> Product/2, Product3/2
  sin/1 -> Product1/1, Product2/2

== system final_fuzzy_modified_fullfuzzy/controller/Subsystem1/triangle finder ==
  In1 : Inport  OutDataType=sfix(16)  OutScaling=2^0
  4 : Gain  Gain=1/60  ParameterDataType=sfix(16)  ParameterScaling=2^0  OutDataType=sfix(16)  OutScaling=2^0
  Rounding Function : Rounding
  Sum15 : Sum  Inputs=|++  OutDataType=sfix(16)  OutScaling=2^0
  Sum7 : Sum  Inputs=|++  OutDataType=sfix(16)  OutScaling=2^0
  Switch : Switch  Criteria=u2 > Threshold  Threshold=-1
  |V|3 : Constant  Value=30  OutDataType=sfix(16)  OutScaling=2^0
  |V|4 : Constant  Value=6  OutDataType=sfix(16)  OutScaling=2^0
  Out1 : Outport  OutDataType=sfix(16)  OutScaling=2^0
  wires:
  |V|3/1 -> Sum7/2
  Sum7/1 -> 4/1
  4/1 -> Rounding Function/1
  Rounding Function/1 -> Switch/2, Switch/1, Sum15/1
  |V|4/1 -> Sum15/2
  Sum15/1 -> Switch/3
  In1/1 -> Sum7/1
  Switch/1 -> Out1/1

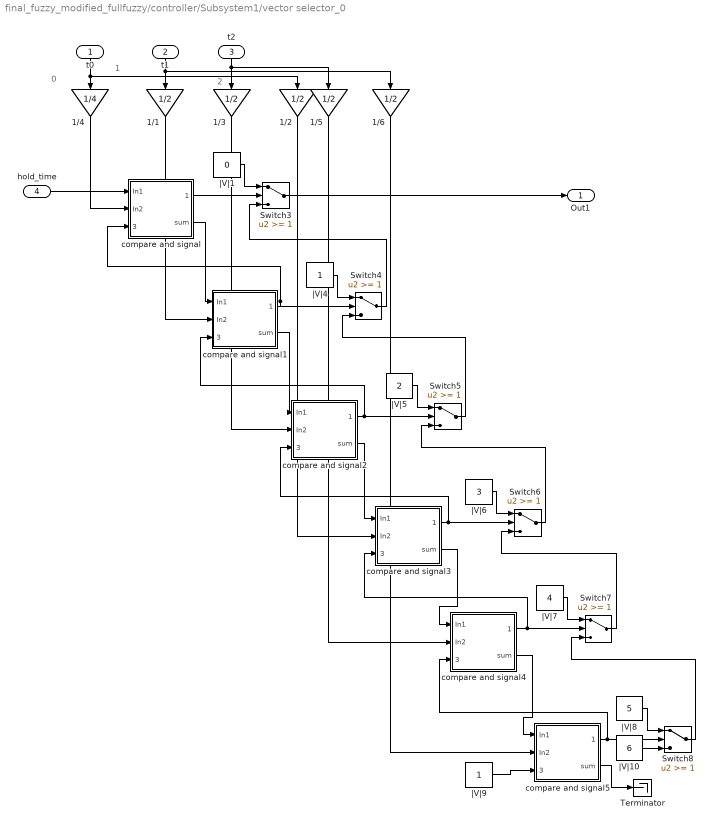
== system final_fuzzy_modified_fullfuzzy/controller/Subsystem1/vector selector_0 ==
  note: 0
  note: 1
  note: 2
  t0 : Inport
  t1 : Inport  Port=2
  t2 : Inport  Port=3
  hold_time : Inport  Port=4
  1/{1..3,5..6} (5 alike) : Gain  Gain=1/2  ParameterDataType=sfix(16)  ParameterScaling=2^0  OutDataType=sfix(16)  OutScaling=2^0
  1/4 : Gain  Gain=1/4  ParameterDataType=sfix(16)  ParameterScaling=2^0  OutDataType=sfix(16)  OutScaling=2^0
  Switch{3..8} (6 alike) : Switch  Threshold=1
  Terminator : Terminator
  compare and signal : Subsystem
  compare and signal1 : Subsystem
  compare and signal2 : Subsystem
  compare and signal3 : Subsystem
  compare and signal4 : Subsystem
  compare and signal5 : Subsystem
  |V|1 : Constant  Value=0  OutDataType=sfix(16)  OutScaling=2^0
  |V|10 : Constant  Value=6  OutDataType=sfix(16)  OutScaling=2^0
  |V|4 : Constant  OutDataType=sfix(16)  OutScaling=2^0
  |V|5 : Constant  Value=2  OutDataType=sfix(16)  OutScaling=2^0
  |V|6 : Constant  Value=3  OutDataType=sfix(16)  OutScaling=2^0
  |V|7 : Constant  Value=4  OutDataType=sfix(16)  OutScaling=2^0
  |V|8 : Constant  Value=5  OutDataType=sfix(16)  OutScaling=2^0
  |V|9 : Constant  OutDataType=sfix(16)  OutScaling=2^0
  Out1 : Outport
  wires:
  1/4/1 -> compare and signal/2(In2)
  t1/1 -> 1/1/1, 1/6/1
  t2/1 -> 1/3/1, 1/5/1
  t0/1 -> 1/4/1, 1/2/1
  hold_time/1 -> compare and signal/1(In1)
  compare and signal/1(logic_out) -> Switch3/2
  |V|1/1 -> Switch3/1
  compare and signal1/1(logic_out) -> compare and signal/3(logic_in), Switch4/2
  compare and signal/2(sum) -> compare and signal1/1(In1)
  1/1/1 -> compare and signal1/2(In2)
  |V|4/1 -> Switch4/1
  compare and signal1/2(sum) -> compare and signal2/1(In1)
  1/3/1 -> compare and signal2/2(In2)
  |V|5/1 -> Switch5/1
  compare and signal2/1(logic_out) -> Switch5/2, compare and signal1/3(logic_in)
  compare and signal2/2(sum) -> compare and signal3/1(In1)
  1/2/1 -> compare and signal3/2(In2)
  |V|6/1 -> Switch6/1
  compare and signal3/1(logic_out) -> Switch6/2, compare and signal2/3(logic_in)
  compare and signal3/2(sum) -> compare and signal4/1(In1)
  1/5/1 -> compare and signal4/2(In2)
  |V|7/1 -> Switch7/1
  compare and signal4/1(logic_out) -> Switch7/2, compare and signal3/3(logic_in)
  1/6/1 -> compare and signal5/2(In2)
  compare and signal4/2(sum) -> compare and signal5/1(In1)
  |V|8/1 -> Switch8/1
  compare and signal5/1(logic_out) -> Switch8/2, compare and signal4/3(logic_in)
  |V|9/1 -> compare and signal5/3(logic_in)
  |V|10/1 -> Switch8/3
  compare and signal5/2(sum) -> Terminator/1
  Switch8/1 -> Switch7/3
  Switch7/1 -> Switch6/3
  Switch6/1 -> Switch5/3
  Switch5/1 -> Switch4/3
  Switch4/1 -> Switch3/3
  Switch3/1 -> Out1/1

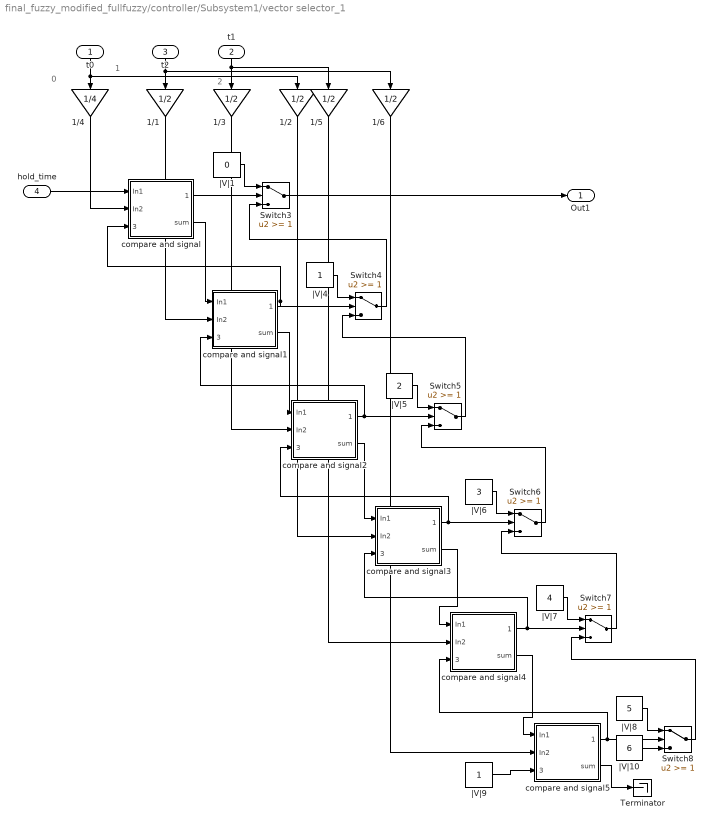
== system final_fuzzy_modified_fullfuzzy/controller/Subsystem1/vector selector_1 ==
  note: 2
  note: 1
  note: 0
  t0 : Inport
  t1 : Inport  Port=2
  t2 : Inport  Port=3
  hold_time : Inport  Port=4
  1/{1..3,5..6} (5 alike) : Gain  Gain=1/2  ParameterDataType=sfix(16)  ParameterScaling=2^0  OutDataType=sfix(16)  OutScaling=2^0
  1/4 : Gain  Gain=1/4  ParameterDataType=sfix(16)  ParameterScaling=2^0  OutDataType=sfix(16)  OutScaling=2^0
  Switch{3..8} (6 alike) : Switch  Threshold=1
  Terminator : Terminator
  compare and signal : Subsystem
  compare and signal1 : Subsystem
  compare and signal2 : Subsystem
  compare and signal3 : Subsystem
  compare and signal4 : Subsystem
  compare and signal5 : Subsystem
  |V|1 : Constant  Value=0  OutDataType=sfix(16)  OutScaling=2^0
  |V|10 : Constant  Value=6  OutDataType=sfix(16)  OutScaling=2^0
  |V|4 : Constant  OutDataType=sfix(16)  OutScaling=2^0
  |V|5 : Constant  Value=2  OutDataType=sfix(16)  OutScaling=2^0
  |V|6 : Constant  Value=3  OutDataType=sfix(16)  OutScaling=2^0
  |V|7 : Constant  Value=4  OutDataType=sfix(16)  OutScaling=2^0
  |V|8 : Constant  Value=5  OutDataType=sfix(16)  OutScaling=2^0
  |V|9 : Constant  OutDataType=sfix(16)  OutScaling=2^0
  Out1 : Outport
  wires:
  Switch3/1 -> Out1/1
  Switch4/1 -> Switch3/3
  Switch5/1 -> Switch4/3
  Switch6/1 -> Switch5/3
  Switch7/1 -> Switch6/3
  Switch8/1 -> Switch7/3
  compare and signal5/2(sum) -> Terminator/1
  |V|10/1 -> Switch8/3
  |V|9/1 -> compare and signal5/3(logic_in)
  compare and signal5/1(logic_out) -> compare and signal4/3(logic_in), Switch8/2
  |V|8/1 -> Switch8/1
  compare and signal4/2(sum) -> compare and signal5/1(In1)
  1/6/1 -> compare and signal5/2(In2)
  compare and signal4/1(logic_out) -> compare and signal3/3(logic_in), Switch7/2
  |V|7/1 -> Switch7/1
  1/5/1 -> compare and signal4/2(In2)
  compare and signal3/2(sum) -> compare and signal4/1(In1)
  compare and signal3/1(logic_out) -> compare and signal2/3(logic_in), Switch6/2
  |V|6/1 -> Switch6/1
  1/2/1 -> compare and signal3/2(In2)
  compare and signal2/2(sum) -> compare and signal3/1(In1)
  compare and signal2/1(logic_out) -> compare and signal1/3(logic_in), Switch5/2
  |V|5/1 -> Switch5/1
  1/3/1 -> compare and signal2/2(In2)
  compare and signal1/2(sum) -> compare and signal2/1(In1)
  |V|4/1 -> Switch4/1
  1/1/1 -> compare and signal1/2(In2)
  compare and signal/2(sum) -> compare and signal1/1(In1)
  compare and signal1/1(logic_out) -> Switch4/2, compare and signal/3(logic_in)
  |V|1/1 -> Switch3/1
  compare and signal/1(logic_out) -> Switch3/2
  hold_time/1 -> compare and signal/1(In1)
  t0/1 -> 1/2/1, 1/4/1
  t1/1 -> 1/5/1, 1/3/1
  t2/1 -> 1/6/1, 1/1/1
  1/4/1 -> compare and signal/2(In2)

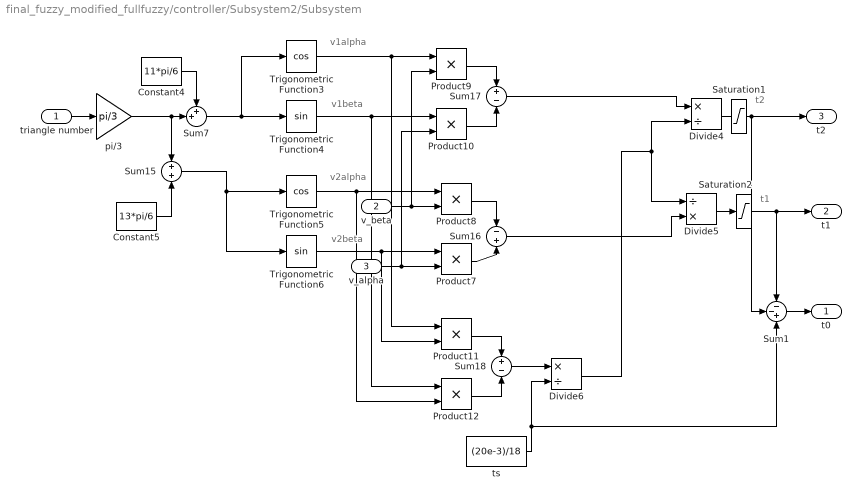
== system final_fuzzy_modified_fullfuzzy/controller/Subsystem2/Subsystem ==
  note: t2
  note: t1
  note: v2beta
  note: v2alpha
  note: v1beta
  note: v1alpha
  triangle number : Inport  OutDataType=sfix(16)  OutScaling=2^0
  v_beta : Inport  Port=2  OutDataType=sfix(16)  OutScaling=2^0
  v_alpha : Inport  Port=3  OutDataType=sfix(16)  OutScaling=2^0
  Constant4 : Constant  Value=11*pi/6  OutDataType=sfix(16)  OutScaling=2^0
  Constant5 : Constant  Value=13*pi/6  OutDataType=sfix(16)  OutScaling=2^0
  Divide4 : Product  Inputs=*/  OutDataType=sfix(16)  OutScaling=2^-10
  Divide5 : Product  Inputs=/*  OutDataType=sfix(16)  OutScaling=2^-10
  Divide6 : Product  Inputs=*/  OutDataType=sfix(16)  OutScaling=2^-10
  Product{7..12} (6 alike) : Product  OutDataType=sfix(16)  OutScaling=2^0  RndMeth=Zero
  Saturation1 : Saturate  UpperLimit=inf  LowerLimit=0
  Saturation2 : Saturate  UpperLimit=inf  LowerLimit=0
  Sum1 : Sum  Inputs=--+  OutDataType=sfix(16)  OutScaling=2^0
  Sum15 : Sum  OutDataType=sfix(16)  OutScaling=2^0
  Sum16 : Sum  Inputs=-+  OutDataType=sfix(16)  OutScaling=2^0
  Sum17 : Sum  Inputs=+-  OutDataType=sfix(16)  OutScaling=2^0
  Sum18 : Sum  Inputs=+-  OutDataType=sfix(16)  OutScaling=2^0
  Sum7 : Sum  Inputs=++|  OutDataType=sfix(16)  OutScaling=2^0
  Trigonometric Function3 : Trigonometry  Operator=cos
  Trigonometric Function4 : Trigonometry
  Trigonometric Function5 : Trigonometry  Operator=cos
  Trigonometric Function6 : Trigonometry
  pi/3 : Gain  Gain=pi/3  ParameterDataType=sfix(16)  ParameterScaling=2^0  OutDataType=sfix(16)  OutScaling=2^0
  ts : Constant  Value=(20e-3)/18  OutDataType=sfix(16)  OutScaling=2^0
  t0 : Outport  OutDataType=sfix(16)  OutScaling=2^0
  t1 : Outport  Port=2  OutDataType=sfix(16)  OutScaling=2^0
  t2 : Outport  Port=3  OutDataType=sfix(16)  OutScaling=2^0
  wires:
  Saturation2/1 -> Sum1/1, t1/1
  Sum1/1 -> t0/1
  Divide5/1 -> Saturation2/1
  triangle number/1 -> pi/3/1
  Divide4/1 -> t2/1, Sum1/2
  v_alpha/1 -> Product10/2, Product7/2
  v_beta/1 -> Product9/2, Product8/2
  ts/1 -> Sum1/3, Divide6/2
  Divide6/1 -> Divide5/1, Divide4/2
  Sum18/1 -> Divide6/1
  Product12/1 -> Sum18/2
  Product11/1 -> Sum18/1
  Sum17/1 -> Divide4/1
  Product10/1 -> Sum17/2
  Product9/1 -> Sum17/1
  Trigonometric Function4/1 -> Product12/1, Product10/1
  Trigonometric Function3/1 -> Product11/1, Product9/1
  Sum16/1 -> Divide5/2
  Product8/1 -> Sum16/1
  Product7/1 -> Sum16/2
  Sum15/1 -> Trigonometric Function6/1, Trigonometric Function5/1
  Trigonometric Function6/1 -> Product11/2, Product7/1
  Trigonometric Function5/1 -> Product12/2, Product8/1
  Constant5/1 -> Sum15/2
  pi/3/1 -> Sum15/1, Sum7/2
  Constant4/1 -> Sum7/1
  Sum7/1 -> Trigonometric Function4/1, Trigonometric Function3/1

== system final_fuzzy_modified_fullfuzzy/controller/Subsystem2/dq to alpha-beta ==
  d : Inport  OutDataType=sfix(16)  OutScaling=2^0
  q : Inport  Port=2  OutDataType=sfix(16)  OutScaling=2^0
  cos : Inport  Port=3  OutDataType=sfix(16)  OutScaling=2^0
  sin : Inport  Port=4  OutDataType=sfix(16)  OutScaling=2^0
  Product{,1..3} (4 alike) : Product  OutDataType=sfix(16)  OutScaling=2^0  RndMeth=Zero
  Sum : Sum  Inputs=+-  OutDataType=sfix(16)  OutScaling=2^0
  Sum1 : Sum  OutDataType=sfix(16)  OutScaling=2^0
  alpha : Outport  OutDataType=sfix(16)  OutScaling=2^0
  beta : Outport  Port=2  OutDataType=sfix(16)  OutScaling=2^0
  wires:
  sin/1 -> Product2/2, Product1/1
  cos/1 -> Product3/2, Product/2
  Sum1/1 -> beta/1
  Product3/1 -> Sum1/2
  Product2/1 -> Sum1/1
  Sum/1 -> alpha/1
  Product1/1 -> Sum/2
  Product/1 -> Sum/1
  q/1 -> Product3/1, Product1/2
  d/1 -> Product2/1, Product/1

== system final_fuzzy_modified_fullfuzzy/controller/Subsystem2/triangle finder ==
  In1 : Inport  OutDataType=sfix(16)  OutScaling=2^0
  4 : Gain  Gain=1/60  ParameterDataType=sfix(16)  ParameterScaling=2^0  OutDataType=sfix(16)  OutScaling=2^0
  Rounding Function : Rounding
  Sum15 : Sum  Inputs=|++  OutDataType=sfix(16)  OutScaling=2^0
  Sum7 : Sum  Inputs=|++  OutDataType=sfix(16)  OutScaling=2^0
  Switch : Switch  Criteria=u2 > Threshold  Threshold=-1
  |V|3 : Constant  Value=30  OutDataType=sfix(16)  OutScaling=2^0
  |V|4 : Constant  Value=6  OutDataType=sfix(16)  OutScaling=2^0
  Out1 : Outport  OutDataType=sfix(16)  OutScaling=2^0
  wires:
  Switch/1 -> Out1/1
  In1/1 -> Sum7/1
  Sum15/1 -> Switch/3
  |V|4/1 -> Sum15/2
  Rounding Function/1 -> Sum15/1, Switch/1, Switch/2
  4/1 -> Rounding Function/1
  Sum7/1 -> 4/1
  |V|3/1 -> Sum7/2

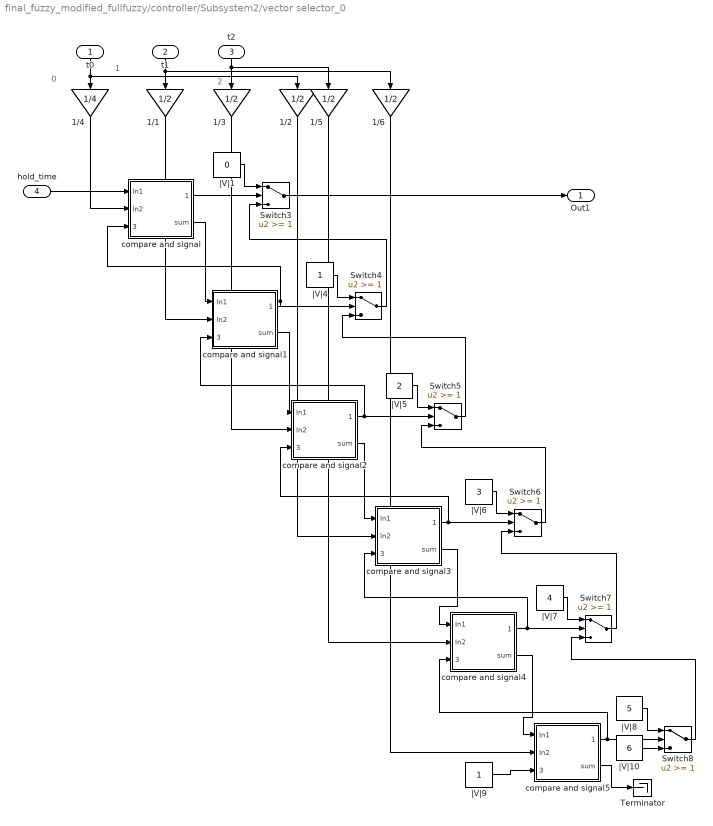
== system final_fuzzy_modified_fullfuzzy/controller/Subsystem2/vector selector_0 ==
  note: 2
  note: 1
  note: 0
  t0 : Inport
  t1 : Inport  Port=2
  t2 : Inport  Port=3
  hold_time : Inport  Port=4
  1/{1..3,5..6} (5 alike) : Gain  Gain=1/2  ParameterDataType=sfix(16)  ParameterScaling=2^0  OutDataType=sfix(16)  OutScaling=2^0
  1/4 : Gain  Gain=1/4  ParameterDataType=sfix(16)  ParameterScaling=2^0  OutDataType=sfix(16)  OutScaling=2^0
  Switch{3..8} (6 alike) : Switch  Threshold=1
  Terminator : Terminator
  compare and signal : Subsystem
  compare and signal1 : Subsystem
  compare and signal2 : Subsystem
  compare and signal3 : Subsystem
  compare and signal4 : Subsystem
  compare and signal5 : Subsystem
  |V|1 : Constant  Value=0  OutDataType=sfix(16)  OutScaling=2^0
  |V|10 : Constant  Value=6  OutDataType=sfix(16)  OutScaling=2^0
  |V|4 : Constant  OutDataType=sfix(16)  OutScaling=2^0
  |V|5 : Constant  Value=2  OutDataType=sfix(16)  OutScaling=2^0
  |V|6 : Constant  Value=3  OutDataType=sfix(16)  OutScaling=2^0
  |V|7 : Constant  Value=4  OutDataType=sfix(16)  OutScaling=2^0
  |V|8 : Constant  Value=5  OutDataType=sfix(16)  OutScaling=2^0
  |V|9 : Constant  OutDataType=sfix(16)  OutScaling=2^0
  Out1 : Outport
  wires:
  Switch3/1 -> Out1/1
  Switch4/1 -> Switch3/3
  Switch5/1 -> Switch4/3
  Switch6/1 -> Switch5/3
  Switch7/1 -> Switch6/3
  Switch8/1 -> Switch7/3
  compare and signal5/2(sum) -> Terminator/1
  |V|10/1 -> Switch8/3
  |V|9/1 -> compare and signal5/3(logic_in)
  compare and signal5/1(logic_out) -> compare and signal4/3(logic_in), Switch8/2
  |V|8/1 -> Switch8/1
  compare and signal4/2(sum) -> compare and signal5/1(In1)
  1/6/1 -> compare and signal5/2(In2)
  compare and signal4/1(logic_out) -> compare and signal3/3(logic_in), Switch7/2
  |V|7/1 -> Switch7/1
  1/5/1 -> compare and signal4/2(In2)
  compare and signal3/2(sum) -> compare and signal4/1(In1)
  compare and signal3/1(logic_out) -> compare and signal2/3(logic_in), Switch6/2
  |V|6/1 -> Switch6/1
  1/2/1 -> compare and signal3/2(In2)
  compare and signal2/2(sum) -> compare and signal3/1(In1)
  compare and signal2/1(logic_out) -> compare and signal1/3(logic_in), Switch5/2
  |V|5/1 -> Switch5/1
  1/3/1 -> compare and signal2/2(In2)
  compare and signal1/2(sum) -> compare and signal2/1(In1)
  |V|4/1 -> Switch4/1
  1/1/1 -> compare and signal1/2(In2)
  compare and signal/2(sum) -> compare and signal1/1(In1)
  compare and signal1/1(logic_out) -> Switch4/2, compare and signal/3(logic_in)
  |V|1/1 -> Switch3/1
  compare and signal/1(logic_out) -> Switch3/2
  hold_time/1 -> compare and signal/1(In1)
  t0/1 -> 1/2/1, 1/4/1
  t2/1 -> 1/5/1, 1/3/1
  t1/1 -> 1/6/1, 1/1/1
  1/4/1 -> compare and signal/2(In2)

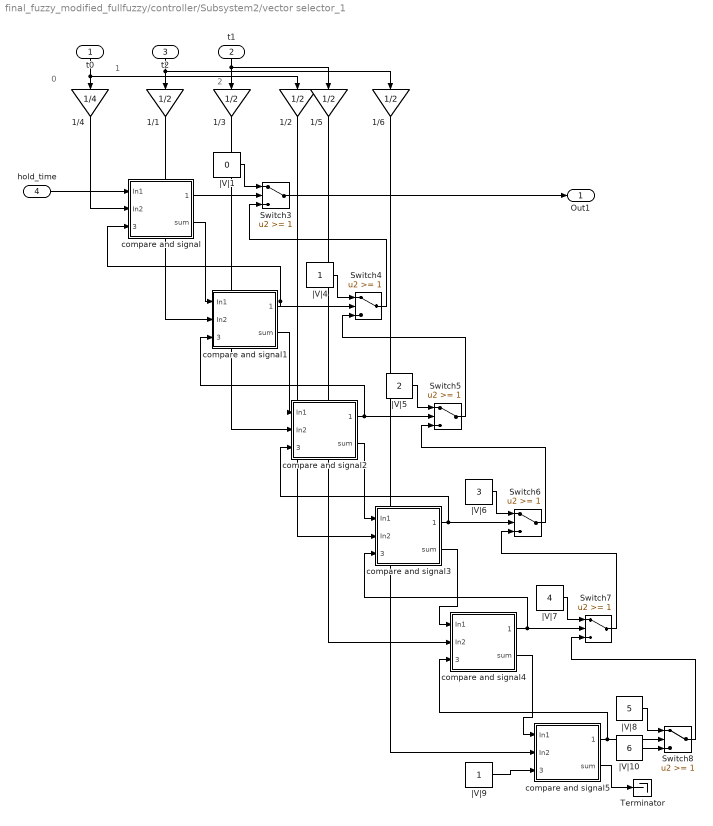
== system final_fuzzy_modified_fullfuzzy/controller/Subsystem2/vector selector_1 ==
  note: 0
  note: 1
  note: 2
  t0 : Inport
  t1 : Inport  Port=2
  t2 : Inport  Port=3
  hold_time : Inport  Port=4
  1/{1..3,5..6} (5 alike) : Gain  Gain=1/2  ParameterDataType=sfix(16)  ParameterScaling=2^0  OutDataType=sfix(16)  OutScaling=2^0
  1/4 : Gain  Gain=1/4  ParameterDataType=sfix(16)  ParameterScaling=2^0  OutDataType=sfix(16)  OutScaling=2^0
  Switch{3..8} (6 alike) : Switch  Threshold=1
  Terminator : Terminator
  compare and signal : Subsystem
  compare and signal1 : Subsystem
  compare and signal2 : Subsystem
  compare and signal3 : Subsystem
  compare and signal4 : Subsystem
  compare and signal5 : Subsystem
  |V|1 : Constant  Value=0  OutDataType=sfix(16)  OutScaling=2^0
  |V|10 : Constant  Value=6  OutDataType=sfix(16)  OutScaling=2^0
  |V|4 : Constant  OutDataType=sfix(16)  OutScaling=2^0
  |V|5 : Constant  Value=2  OutDataType=sfix(16)  OutScaling=2^0
  |V|6 : Constant  Value=3  OutDataType=sfix(16)  OutScaling=2^0
  |V|7 : Constant  Value=4  OutDataType=sfix(16)  OutScaling=2^0
  |V|8 : Constant  Value=5  OutDataType=sfix(16)  OutScaling=2^0
  |V|9 : Constant  OutDataType=sfix(16)  OutScaling=2^0
  Out1 : Outport
  wires:
  1/4/1 -> compare and signal/2(In2)
  t2/1 -> 1/1/1, 1/6/1
  t1/1 -> 1/3/1, 1/5/1
  t0/1 -> 1/4/1, 1/2/1
  hold_time/1 -> compare and signal/1(In1)
  compare and signal/1(logic_out) -> Switch3/2
  |V|1/1 -> Switch3/1
  compare and signal1/1(logic_out) -> compare and signal/3(logic_in), Switch4/2
  compare and signal/2(sum) -> compare and signal1/1(In1)
  1/1/1 -> compare and signal1/2(In2)
  |V|4/1 -> Switch4/1
  compare and signal1/2(sum) -> compare and signal2/1(In1)
  1/3/1 -> compare and signal2/2(In2)
  |V|5/1 -> Switch5/1
  compare and signal2/1(logic_out) -> Switch5/2, compare and signal1/3(logic_in)
  compare and signal2/2(sum) -> compare and signal3/1(In1)
  1/2/1 -> compare and signal3/2(In2)
  |V|6/1 -> Switch6/1
  compare and signal3/1(logic_out) -> Switch6/2, compare and signal2/3(logic_in)
  compare and signal3/2(sum) -> compare and signal4/1(In1)
  1/5/1 -> compare and signal4/2(In2)
  |V|7/1 -> Switch7/1
  compare and signal4/1(logic_out) -> Switch7/2, compare and signal3/3(logic_in)
  1/6/1 -> compare and signal5/2(In2)
  compare and signal4/2(sum) -> compare and signal5/1(In1)
  |V|8/1 -> Switch8/1
  compare and signal5/1(logic_out) -> Switch8/2, compare and signal4/3(logic_in)
  |V|9/1 -> compare and signal5/3(logic_in)
  |V|10/1 -> Switch8/3
  compare and signal5/2(sum) -> Terminator/1
  Switch8/1 -> Switch7/3
  Switch7/1 -> Switch6/3
  Switch6/1 -> Switch5/3
  Switch5/1 -> Switch4/3
  Switch4/1 -> Switch3/3
  Switch3/1 -> Out1/1

== system final_fuzzy_modified_fullfuzzy/controller/Subsystem3/Fuzzy Logic  Controller ==
  In1 : Inport  OutDataType=sfix(16)  OutScaling=2^0
  Demux : Demux  Outputs=2
  FIS Wizard : fuzwiz/FIS Wizard  SystemSampleTime=-1  fis=fis
  PI5 : Subsystem
  Out1 : Outport  OutDataType=sfix(16)  OutScaling=2^0
  wires:
  PI5/1(Out1) -> Out1/1
  In1/1 -> Demux/1
  Demux/1 -> PI5/1(In1)

== system final_fuzzy_modified_fullfuzzy/controller/Subsystem4/Fuzzy Logic  Controller ==
  In1 : Inport  OutDataType=sfix(16)  OutScaling=2^0
  Demux : Demux  Outputs=2
  FIS Wizard : fuzwiz/FIS Wizard  SystemSampleTime=-1  fis=fis
  PI2 : Subsystem
  Out1 : Outport  OutDataType=sfix(16)  OutScaling=2^0
  wires:
  In1/1 -> Demux/1
  PI2/1(Out1) -> Out1/1
  Demux/1 -> PI2/1(In1)

== system final_fuzzy_modified_fullfuzzy/controller/Subsystem5/Fuzzy Logic  Controller ==
  In1 : Inport  OutDataType=sfix(16)  OutScaling=2^0
  Demux : Demux  Outputs=2
  FIS S-function : S-Function  FunctionName=sffis  Parameters=fis  SFunctionModules=sfsup  EnableBusSupport=off
  PI1 : Subsystem
  Out1 : Outport  OutDataType=sfix(16)  OutScaling=2^0
  wires:
  Demux/1 -> PI1/1(In1)
  In1/1 -> Demux/1
  PI1/1(Out1) -> Out1/1

== system final_fuzzy_modified_fullfuzzy/controller/Subsystem1/vector selector_0/compare and signal ==
  In1 : Inport
  In2 : Inport  Port=2
  logic_in : Inport  Port=3
  " 2" : Logic  AllPortsSameDT=off  OutDataTypeMode=boolean  OutDataTypeStr=boolean
  Clock1 : Clock
      settings: Decimation=10
  Relational Operator3 : RelationalOperator  LogicOutDataTypeMode=boolean  OutDataTypeStr=boolean
  Sum1 : Sum  Inputs=++|  OutDataType=sfix(16)  OutScaling=2^0
  logic_out : Outport
  sum : Outport  Port=2
  wires:
  Sum1/1 -> Relational Operator3/1, sum/1
  Clock1/1 -> Relational Operator3/2
  Relational Operator3/1 -> " 2"/1
  In1/1 -> Sum1/1
  In2/1 -> Sum1/2
  " 2"/1 -> logic_out/1
  logic_in/1 -> " 2"/2

== system final_fuzzy_modified_fullfuzzy/controller/Subsystem1/vector selector_0/compare and signal1 ==
  In1 : Inport
  In2 : Inport  Port=2
  logic_in : Inport  Port=3
  " 2" : Logic  AllPortsSameDT=off  OutDataTypeMode=boolean  OutDataTypeStr=boolean
  Clock1 : Clock
      settings: Decimation=10
  Relational Operator3 : RelationalOperator  LogicOutDataTypeMode=boolean  OutDataTypeStr=boolean
  Sum1 : Sum  Inputs=++|  OutDataType=sfix(16)  OutScaling=2^0
  logic_out : Outport
  sum : Outport  Port=2
  wires:
  logic_in/1 -> " 2"/2
  " 2"/1 -> logic_out/1
  In2/1 -> Sum1/2
  In1/1 -> Sum1/1
  Relational Operator3/1 -> " 2"/1
  Clock1/1 -> Relational Operator3/2
  Sum1/1 -> sum/1, Relational Operator3/1

== system final_fuzzy_modified_fullfuzzy/controller/Subsystem1/vector selector_0/compare and signal2 ==
  In1 : Inport
  In2 : Inport  Port=2
  logic_in : Inport  Port=3
  " 2" : Logic  AllPortsSameDT=off  OutDataTypeMode=boolean  OutDataTypeStr=boolean
  Clock1 : Clock
      settings: Decimation=10
  Relational Operator3 : RelationalOperator  LogicOutDataTypeMode=boolean  OutDataTypeStr=boolean
  Sum1 : Sum  Inputs=++|  OutDataType=sfix(16)  OutScaling=2^0
  logic_out : Outport
  sum : Outport  Port=2
  wires:
  Sum1/1 -> Relational Operator3/1, sum/1
  Clock1/1 -> Relational Operator3/2
  Relational Operator3/1 -> " 2"/1
  In1/1 -> Sum1/1
  In2/1 -> Sum1/2
  " 2"/1 -> logic_out/1
  logic_in/1 -> " 2"/2
